simulink model "Exercitiul5"  (R2016a)
settings: Solver=VariableStepDiscrete  StartTime=0.0  StopTime=60  RelTol=1e-3
undefined symbols (not defined in the file): m, n
settings Model: Creator=Cristina  LastModifiedBy=Cristina

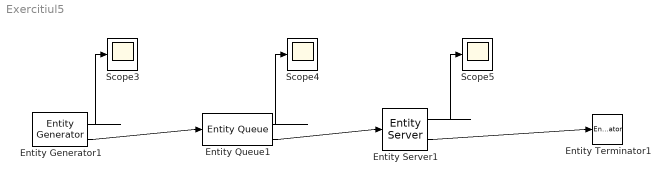
== system Exercitiul5 ==
  Entity Generator1 : EntityGenerator  OutputPortMessageModes=n,m  TimeSource=MATLAB action  IntergenerationTimeAction=dt = exprnd(0.1);  NumberEntitiesDeparted=on  EntityType=Structured  EntityTypeName=Entity
      settings: OutputPortMap=o0,o3
  Entity Queue1 : EntityQueue  InputPortMessageModes=m  OutputPortMessageModes=n,m  AverageWait=on
      settings: OutputPortMap=o2,o5
  Entity Server1 : EntityServer  InputPortMessageModes=m  OutputPortMessageModes=n,m  ServiceTimeSource=MATLAB action  ServiceTimeAction=|  NumberEntitiesDeparted=on
      | presistent init
      | if (isempty(init))
      |     rng(155);
      |     init = true;
      | end
      | dt = (1.2-0.8) * rand + 0.8
      settings: OutputPortMap=o0,o9
  Entity Terminator1 : EntityTerminator  InputPortMessageModes=m
  Scope3 : Scope
  Scope4 : Scope
  Scope5 : Scope
  wires:
  Entity Generator1/2 -> Entity Queue1/1
  Entity Queue1/2 -> Entity Server1/1
  Entity Server1/2 -> Entity Terminator1/1
  Entity Generator1/1 -> Scope3/1
  Entity Server1/1 -> Scope5/1
  Entity Queue1/1 -> Scope4/1
